simulink model "nxtway_gs_plant"  (Simulink 7.0)
settings: Solver=ode45  StartTime=0.0  StopTime=10.0  MaxStep=TS  RelTol=1e-3
PreLoadFcn:
  | param_nxtway_gs
values from neighbouring files (symbols this model uses):
  A1 = [ ... (first row only)    [param_plant.m]
  A2 = [ ... (first row only)    [param_plant.m]
  B1 = [ ... (first row only)    [param_plant.m]
  B2 = [ ... (first row only)    [param_plant.m]
  C1 = eye(4)    [param_plant.m]
  C2 = eye(2)    [param_plant.m]
  D1 = zeros(4, 2)    [param_plant.m]
  D2 = zeros(2)    [param_plant.m]
  X1IV = [ ... (first row only)    [param_sim.m]
  X2IV = [ ... (first row only)    [param_sim.m]
settings Model: Creator=y_yama  LastModifiedBy=y_yama
settings DataIOCC: SaveOutput=off  SignalLogging=off  SaveTime=off
settings OptimizationCC: InlineParams=on  InlineInvariantSignals=on  LifeSpan=1
settings HardwareCC: ProdIntDivRoundTo=Zero  ProdEndianess=LittleEndian  ProdHWDeviceType=ARM Compatible->ARM 7

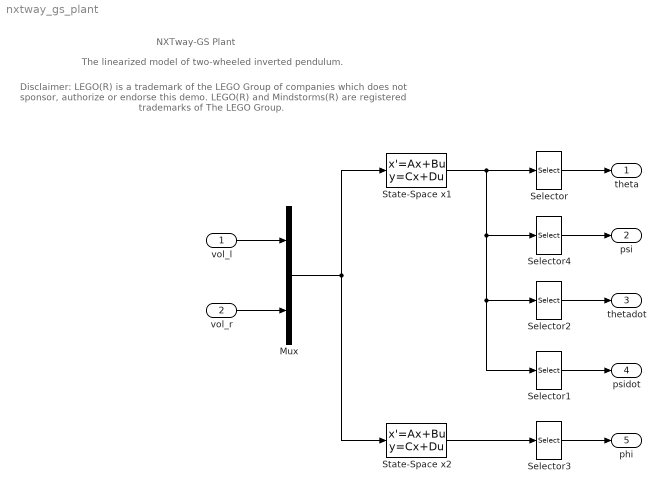
== system nxtway_gs_plant ==
  note: NXTway-GS Plant
  note: The linearized model of two-wheeled inverted pendulum.
  note: Disclaimer:
      | LEGO(R) is a trademark of the LEGO Group of companies which does not sponsor,
      | authorize or endorse this demo.
      | LEGO(R) and Mindstorms(R) are registered trademarks of The LEGO Group.
  vol_l : Inport  DataType=double  OutDataType=sfix(16)  OutScaling=2^0
  vol_r : Inport  Port=2  DataType=double  OutDataType=sfix(16)  OutScaling=2^0
  Mux : Mux  Inputs=2
  Selector : Selector  InputPortWidth=4  IndexOptions=Index vector (dialog)  Indices=1  OutputSizes=1
  Selector1 : Selector  InputPortWidth=4  IndexOptions=Index vector (dialog)  Indices=4  OutputSizes=1
  Selector2 : Selector  InputPortWidth=4  IndexOptions=Index vector (dialog)  Indices=3  OutputSizes=1
  Selector3 : Selector  InputPortWidth=2  IndexOptions=Index vector (dialog)  Indices=1  OutputSizes=1
  Selector4 : Selector  InputPortWidth=4  IndexOptions=Index vector (dialog)  Indices=2  OutputSizes=1
  State-Space x1 : StateSpace  A=A1  B=B1  C=C1  D=D1  X0=X1IV
  State-Space x2 : StateSpace  A=A2  B=B2  C=C2  D=D2  X0=X2IV
  theta : Outport  OutDataType=sfix(16)  OutScaling=2^0
  psi : Outport  Port=2  OutDataType=sfix(16)  OutScaling=2^0
  thetadot : Outport  Port=3  OutDataType=sfix(16)  OutScaling=2^0
  psidot : Outport  Port=4  OutDataType=sfix(16)  OutScaling=2^0
  phi : Outport  Port=5  OutDataType=sfix(16)  OutScaling=2^0
  wires:
  vol_l/1 -> Mux/1
  vol_r/1 -> Mux/2
  Mux/1 -> State-Space x1/1, State-Space x2/1
  State-Space x1/1 -> Selector/1, Selector2/1, Selector1/1, Selector4/1
  State-Space x2/1 -> Selector3/1
  Selector/1 -> theta/1
  Selector3/1 -> phi/1
  Selector2/1 -> thetadot/1
  Selector1/1 -> psidot/1
  Selector4/1 -> psi/1
